simulink model "AM"  (R2018b)
settings: Solver=VariableStepAuto  StartTime=0.0  StopTime=10.0  RelTol=1e-3
libraries: commanapbnd3 x1
settings Model: Creator=sin  LastModifiedBy=sin

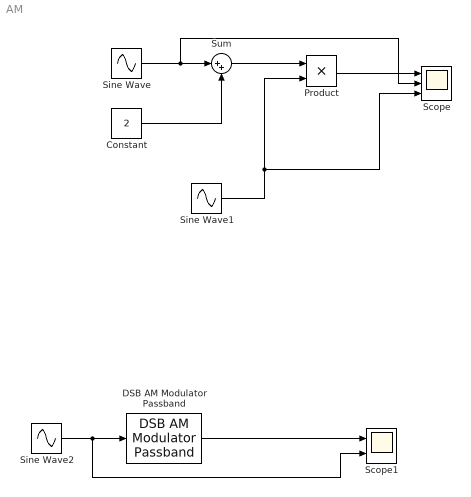
== system AM ==
  Constant : Constant  Value=2
  DSB AM Modulator Passband : commanapbnd3/DSB AM Modulator Passband  Fc=10  Ph=0  Offset=1
      settings: SourceProductName=Communications System Toolbox  SourceProductBaseCode=CM
  Product : Product
  Scope : Scope  NumInputPorts=3
  Scope1 : Scope  NumInputPorts=2
  Sine Wave : Sin  Frequency=1*2*pi  SampleTime=0
  Sine Wave1 : Sin  Frequency=10*2*pi  SampleTime=0
  Sine Wave2 : Sin  Frequency=1*2*pi  SampleTime=0.001
  Sum : Sum  Inputs=|++
  wires:
  Sine Wave/1 -> Scope/2, Sum/1
  Constant/1 -> Sum/2
  Sum/1 -> Product/1
  Sine Wave1/1 -> Scope/3, Product/2
  Product/1 -> Scope/1
  Sine Wave2/1 -> Scope1/2, DSB AM Modulator Passband/1
  DSB AM Modulator Passband/1 -> Scope1/1
